simulink library "hapsrav_library"  (R2017a)
settings: Solver=VariableStepAuto  StartTime=0.0  StopTime=10.0  RelTol=1e-3
values from neighbouring files (symbols this model uses):
  absorb_h = 0:100:40000    [EnergySim.m]
  Adisk = pi * v.R_prop^2    [EnergySim.m]
  alpha_h = absorb_h    [EnergySim.m]
  aoa_data = zeros(n_cl, n)    [EnergySim.m]
  cl_bp = linspace(min_cl, max_cl,n_cl)    [EnergySim.m]
  D = [1       -.0065      288.15          0                   101325 ... (first row only)    [EnergySim.m]    (also in msn_params.m = sqrt((from_x - to_x)^2 + (from_y - to_y)^2); solar_vector.m = time.day + ut_time)
  d2r = pi / 180    (= 0.0174532925199)    [EnergySim.m]    (also in example1.m; example2.m; example3.m; example4.m)
  d_init = sqrt(dx*dx + dy*dy)    [EnergySim.m]    (also in msn_init.m)
  dchi0 = atan2(sin(dchi0), cos(dchi0))    [EnergySim.m]    (also in msn_init.m)
  dT = 0.5    [EnergySim.m]
  dT_fixed = 0.5    [EnergySim.m]
  dT_trig = 30    [EnergySim.m]
  earth_rho = 6378137.0    (= 6378137)    [EnergySim.m]
  fp = solarFP(p.orbit_rho, p.min_axis, p.orbit_dir, ic.x_ctr, ic.y_ctr, sun_az_0)    [EnergySim.m]    (also in load_fp.m = gid_tc(msn_idx).fp; solarFP.m = [1	6	2	nul eul 0	0	0	0	1	0)
  fp_coords = [x_entry y_entry]    [msn_params.m]
  fp_courses = [chi_adj nxt_chi dchi]    [msn_params.m]
  g = 9.80665    [EnergySim.m]
  Gsolar = 1367    [EnergySim.m]
  k = k+1    (= 5)    [EnergySim.m]
  K = D(:,2)    [EnergySim.m]
  lat_init = ic.lat_init_deg * obj.d2r    [EnergySim.m]
  M = time.month    [solar_vector.m]
  max_cl = max(cl_data(:))    [EnergySim.m]
  min_cl = min(cl_data(:))    [EnergySim.m]
  ND2 = load(fullfile(pwd,'nd2_data.mat'))    [EnergySim.m]    (also in nd2_data.mat = [0.0999999999999 0.200000000001 0.3 0.4 0.499999999998 0.700)
  next_init = fp(init_wp, 3)    [EnergySim.m]    (also in msn_init.m)
  pE_init = ic.pE_init    [EnergySim.m]
  pN_init = ic.pN_init    [EnergySim.m]
  r2d = 180 / pi    (= 57.2957795131)    [EnergySim.m]    (also in example1.m; example2.m; example3.m; example4.m)
  rho_SL = 1.225    [EnergySim.m]
  S = 110.4    [EnergySim.m]
  thr_lo_lim = 0.0    (= 0)    [EnergySim.m]
  time_init = struct('year', time.year, 'month', time.month,                  'day', time.day, 'hour', time.hour, 'min', time.min,                  'UTC', time.UTC)    [EnergySim.m]
  to_init = fp(init_wp, 1)    [EnergySim.m]    (also in msn_init.m)
  vgnd_init = sqrt(Vg)    [EnergySim.m]
  vtas_init = veas_init * sqrt(rho_sl/rho_alt)    [EnergySim.m]
  w_alt = 2.0 * w_alt    [EnergySim.m]
  w_xtrack = 2.0 * w_xtrack    [EnergySim.m]
undefined symbols (not defined in the file or in its folder): alpha, alpha_bp, alpha_circ, alt0_rate_init, alt_bp, alt_cmd_mode, alt_init, alt_lim_h, alt_lim_l, alt_rt_lim_periodic, cd_data, charge_eff, chi0_rate_init, chi_cmd_mode, chi_inf, chi_init, cl_data, discharge_eff, DiscIntNeverNeededParam, E_batt_max, E_init, Earth, enableFuzzyLogic, entry_init, epsln, epsln_circ, exit_init, f8_azimuth_offset, fig_eight_time, fp0, fp_coords0, fp_courses0, gamma_lim, hold_time, k_c, K_circ, lat_init_deg, lon_init_deg, max_alpha_bp, max_alt_bp, min_alpha_bp, min_alt_bp, min_axis, motor_eff, mppt_eff, num_motors, orb_dir_init, orb_len_init, orbit_dir, orbit_rho, P_acc, panel_eff, panel_vecs, phi_0, phi_lim, phi_lim_alt, phi_lim_alt_max, phi_lim_alt_min, phi_rt_lim, prop_eff_scale ... (+39)
libraries: simulink x59, hapsrav_library x9, fuzblock x3, atmospheric_library x1, aerolibtransform2 x1
(part 3 of 6)

== system hapsrav_library/hapsrav_main/Kinematic 6DOF/Aero/Thrust ==
  d1Vtas : Inport
  gamma : Inport  Port=2
  qS : Inport  Port=3
  CL : Inport  Port=4
  CD : Inport  Port=5
  Display1 : Display
  Display2 : Display
  Display3 : Display
  Divide : Product  Inputs=**
  Divide1 : Product  Inputs=**
  Gain1 : Gain  Gain=M*g
  Gain2 : Gain  Gain=M
  Saturation : Saturate  UpperLimit=9999  LowerLimit=thr_lo_lim
  Sum1 : Sum  Inputs=|++
  Sum5 : Sum  Inputs=|++
  Terminator : Terminator
  Terminator1 : Terminator
  Trigonometric Function : Trigonometry
  thrust : Outport
  wires:
  Saturation/1 -> [thrust]
  Gain1/1 -> Sum1/2
  d1Vtas/1 -> Gain2/1
  Gain2/1 -> Sum1/1
  CL/1 -> Divide/1
  qS/1 -> [qS]
  [qS] -> Divide/2
  Divide/1 -> Display3/1, [lift]
  gamma/1 -> [gamma]
  [gamma] -> Trigonometric Function/1
  Trigonometric Function/1 -> [sin_gamma]
  [sin_gamma] -> Gain1/1
  Sum1/1 -> Sum5/1
  [drag] -> Sum5/2, Display2/1
  [qS] -> Divide1/2
  Divide1/1 -> [drag]
  Sum5/1 -> Display1/1, thrust/1, Saturation/1
  CD/1 -> Divide1/1
  [lift] -> Terminator/1
  [thrust] -> Terminator1/1

== system hapsrav_library/hapsrav_main/Kinematic 6DOF/Airspeed/Std Atmos ==
  alt : Inport
  Constant : Constant  Value=rho_SL
  Divide : Product  Inputs=*/
  NASA-TM-X-74335 Std Atmos 1976 -5 < Alt < 47 km : atmospheric_library/NASA-TM-X-74335 Std Atmos 1976 -5 < Alt < 47 km
  Sqrt : Sqrt  SaturateOnIntegerOverflow=on
  Terminator : Terminator
  rho_ratio : Outport
  OAT : Outport  Port=2
  wires:
  [stat_press] -> Terminator/1
  alt/1 -> NASA-TM-X-74335 Std Atmos 1976 -5 < Alt < 47 km/1
  NASA-TM-X-74335 Std Atmos 1976 -5 < Alt < 47 km/3 -> [rho]
  NASA-TM-X-74335 Std Atmos 1976 -5 < Alt < 47 km/1 -> [OAT]
  NASA-TM-X-74335 Std Atmos 1976 -5 < Alt < 47 km/2 -> [stat_press]
  [OAT] -> OAT/1
  Sqrt/1 -> rho_ratio/1
  Divide/1 -> Sqrt/1
  [rho] -> Divide/2
  Constant/1 -> Divide/1

== system hapsrav_library/hapsrav_main/Kinematic 6DOF/Inertial/East Wind Error ==
  In1 : Inport
  In2 : Inport  Port=2
  In3 : Inport  Port=3
  In4 : Inport  Port=4
  In5 : Inport  Port=5
  In6 : Inport  Port=6
  In7 : Inport  Port=7
  Divide12 : Product  Inputs=***
  Divide13 : Product  Inputs=***
  Sum8 : Sum  Inputs=|+-
  Sum9 : Sum  Inputs=+-|
  We Error : Outport
  wires:
  In4/1 -> Divide12/3
  In2/1 -> Divide12/1
  Divide12/1 -> Sum8/1
  Divide13/1 -> Sum8/2
  In5/1 -> Divide13/1
  In6/1 -> Divide13/2
  In3/1 -> Divide12/2
  In1/1 -> Sum9/1
  Sum9/1 -> We Error/1
  In7/1 -> Divide13/3
  Sum8/1 -> Sum9/2

== system hapsrav_library/hapsrav_main/Kinematic 6DOF/Inertial/Gnd Speed ==
  note: Equation (2.12) of small unmanned aircraft, R. Beard, T. McLain
  Vw2 : Inport
  Vtas : Inport  Port=2
  cos_psi : Inport  Port=3
  cos_ga : Inport  Port=4
  wn : Inport  Port=5
  sin_psi : Inport  Port=6
  we : Inport  Port=7
  sin_ga : Inport  Port=8
  wd : Inport  Port=9
  vgnd0 : Inport  Port=10
  Constant : Constant  Value=0
  Delay2 : Delay  DelayLength=1  InitialConditionSource=Input port
      settings: InputPortMap=u0,p4
  Discrete Differentiator1 : hapsrav_library/Discrete Differentiator
  Divide5 : Product  Inputs=***
  Divide7 : Product  Inputs=***
  Divide8 : Product  Inputs=**
  Divide9 : Product  Inputs=**
  Gain : Gain  Gain=2
  Math Function3 : Math  Operator=square  SaturateOnIntegerOverflow=on
  Sqrt : Sqrt  SaturateOnIntegerOverflow=on
  Sum1 : Sum  Inputs=|++
  Sum4 : Sum  Inputs=+++
  Sum5 : Sum  Inputs=|+-
  Vg : Outport
  d1Vg : Outport  Port=2
  wires:
  Constant/1 -> Discrete Differentiator1/3
  Math Function3/1 -> Sum4/2
  wn/1 -> Divide5/3
  sin_psi/1 -> Divide7/1
  sin_ga/1 -> Divide8/1
  wd/1 -> Divide8/2
  we/1 -> Divide7/3
  cos_psi/1 -> Divide5/1
  Vw2/1 -> Sum4/1
  Gain/1 -> Divide9/1
  Sum4/1 -> Sqrt/1
  Divide9/1 -> Sum4/3
  cos_ga/1 -> [cos_ga]
  [cos_ga] -> Divide5/2
  [cos_ga] -> Divide7/2
  Vtas/1 -> [Vtas]
  [Vtas] -> Gain/1
  [Vtas] -> Math Function3/1
  Divide5/1 -> Sum1/1
  Divide7/1 -> Sum1/2
  Sum1/1 -> Sum5/1
  Divide8/1 -> Sum5/2
  Sum5/1 -> Divide9/2
  Discrete Differentiator1/1 -> d1Vg/1
  Delay2/1 -> Discrete Differentiator1/1, Vg/1
  vgnd0/1 -> Discrete Differentiator1/2, Delay2/2
  Sqrt/1 -> Delay2/1

== system hapsrav_library/hapsrav_main/Kinematic 6DOF/Inertial/Heading ==
  note: Equation (2.11) of small unmanned aircraft, R. Beard, T. McLain
  wn : Inport
  sin_chi : Inport  Port=2
  cos_chi : Inport  Port=3
  we : Inport  Port=4
  Vtas : Inport  Port=5
  cos_ga : Inport  Port=6
  chi : Inport  Port=7
  Divide2 : Product  Inputs=**
  Divide3 : Product  Inputs=**
  Divide4 : Product  Inputs=*/
  Divide6 : Product  Inputs=**
  Sum1 : Sum  Inputs=|-+
  Sum2 : Sum  Inputs=|-+
  Trigonometric Function5 : Trigonometry  Operator=asin
  psi : Outport
  wires:
  we/1 -> Divide3/2
  Divide2/1 -> Sum1/1
  wn/1 -> Divide2/1
  cos_ga/1 -> Divide6/2
  Divide6/1 -> Divide4/2
  Divide4/1 -> Trigonometric Function5/1
  Trigonometric Function5/1 -> Sum2/1
  Divide3/1 -> Sum1/2
  Sum1/1 -> Divide4/1
  Vtas/1 -> Divide6/1
  Sum2/1 -> psi/1
  chi/1 -> Sum2/2
  cos_chi/1 -> Divide3/1
  sin_chi/1 -> Divide2/2

== system hapsrav_library/hapsrav_main/Kinematic 6DOF/Inertial/North Wind Error ==
  In1 : Inport
  In2 : Inport  Port=2
  In3 : Inport  Port=3
  In4 : Inport  Port=4
  In5 : Inport  Port=5
  In6 : Inport  Port=6
  In7 : Inport  Port=7
  Divide10 : Product  Inputs=***
  Divide11 : Product  Inputs=***
  Sum6 : Sum  Inputs=|+-
  Sum7 : Sum  Inputs=+-|
  Wn Error : Outport
  wires:
  In7/1 -> Divide11/3
  In1/1 -> Sum7/1
  Divide10/1 -> Sum6/1
  Divide11/1 -> Sum6/2
  In4/1 -> Divide10/3
  In3/1 -> Divide10/2
  In6/1 -> Divide11/2
  Sum6/1 -> Sum7/2
  In5/1 -> Divide11/1
  In2/1 -> Divide10/1
  Sum7/1 -> Wn Error/1

== system hapsrav_library/hapsrav_main/Kinematic 6DOF/Navigation/Flat Earth to LLA ==
  lat0 : Inport
  lon0 : Inport  Port=2
  pos_N_dot : Inport  Port=3
  pos_E_dot : Inport  Port=4
  alt : Inport  Port=5
  Discrete-Time Integrator : DiscreteIntegrator  IntegratorMethod=Integration: Trapezoidal  InitialConditionSource=external  InitialConditionSetting=State (most efficient)  SampleTime=dT  ICPrevOutput=DiscIntNeverNeededParam  ICPrevScaledInput=DiscIntNeverNeededParam
  Discrete-Time Integrator1 : DiscreteIntegrator  IntegratorMethod=Integration: Trapezoidal  InitialConditionSource=external  InitialConditionSetting=State (most efficient)  SampleTime=dT  ICPrevOutput=DiscIntNeverNeededParam  ICPrevScaledInput=DiscIntNeverNeededParam
  Divide : Product  Inputs=*/
  Divide1 : Product  Inputs=**
  Divide2 : Product  Inputs=*/
  Memory : Memory  X0=lat_init
  Radii of Curvature : Subsystem
  Trigonometric Function1 : Trigonometry  Operator=cos
  wn^1 : Gain  Gain=r2d
  wn^2 : Gain  Gain=r2d
  lat_est : Outport
  lon_est : Outport  Port=2
  wires:
  Radii of Curvature/2(R_M) -> [R_M]
  Radii of Curvature/1(R_N) -> [R_N]
  [lat_est] -> Trigonometric Function1/1
  wn^2/1 -> lat_est/1
  wn^1/1 -> lon_est/1
  [lat_est] -> Memory/1
  Divide/1 -> Discrete-Time Integrator/1
  [R_M] -> Divide/2
  Discrete-Time Integrator/1 -> [lat_est], wn^2/1
  pos_N_dot/1 -> Divide/1
  Discrete-Time Integrator1/1 -> wn^1/1
  pos_E_dot/1 -> Divide2/1
  lat0/1 -> Discrete-Time Integrator/2
  lon0/1 -> Discrete-Time Integrator1/2
  Memory/1 -> Radii of Curvature/1(lat_rad)
  [R_N] -> Divide1/2
  Trigonometric Function1/1 -> Divide1/1
  Divide2/1 -> Discrete-Time Integrator1/1
  Divide1/1 -> Divide2/2
  alt/1 -> [alt]
  [alt] -> Radii of Curvature/2(h)

== system hapsrav_library/hapsrav_main/Kinematic 6DOF/Navigation/Flat Earth to LLA Aero BLockset ==
  alt : Inport
  pN : Inport  Port=2
  pE : Inport  Port=3
  Demux : Demux  Outputs=2
  Flat Earth to LLA : aerolibtransform2/Flat Earth to LLA  units=Metric (MKS)  ptype=Earth (WGS84)  F=1/298.257223563  R=6378137  LL0=[lat_init_deg lon_init_deg]  psi=0
  Mux : Mux  Inputs=3
  Ref Alt : Constant  Value=0
  Terminator : Terminator
  wn^3 : Gain  Gain=-1
  lat_deg : Outport
  lon_deg : Outport  Port=2
  wires:
  wn^3/1 -> Mux/3
  Ref Alt/1 -> Flat Earth to LLA/2
  Mux/1 -> Flat Earth to LLA/1
  alt/1 -> wn^3/1
  pE/1 -> Mux/2
  pN/1 -> Mux/1
  Demux/1 -> lat_deg/1
  Demux/2 -> lon_deg/1
  Flat Earth to LLA/2 -> Terminator/1
  Flat Earth to LLA/1 -> Demux/1

== system hapsrav_library/hapsrav_main/Kinematic 6DOF/Navigation/NED Posn ==
  note: Equation (9.8) of small unmanned aircraft, R. Beard, T. McLain
  Va : Inport
  psi : Inport  Port=2
  we : Inport  Port=3
  wn : Inport  Port=4
  pE0 : Inport  Port=5
  pN0 : Inport  Port=6
  Discrete-Time Integrator : DiscreteIntegrator  IntegratorMethod=Integration: Trapezoidal  InitialConditionSource=external  InitialConditionSetting=State (most efficient)  SampleTime=-1  ICPrevOutput=DiscIntNeverNeededParam  ICPrevScaledInput=DiscIntNeverNeededParam
  Discrete-Time Integrator1 : DiscreteIntegrator  IntegratorMethod=Integration: Trapezoidal  InitialConditionSource=external  InitialConditionSetting=State (most efficient)  SampleTime=-1  ICPrevOutput=DiscIntNeverNeededParam  ICPrevScaledInput=DiscIntNeverNeededParam
  Divide : Product
  Divide1 : Product
  Sum1 : Sum  Inputs=|++
  Sum2 : Sum  Inputs=|++
  Trigonometric Function : Trigonometry
  Trigonometric Function1 : Trigonometry  Operator=cos
  pE : Outport
  pE_dot : Outport  Port=2
  pN : Outport  Port=3
  pN_dot : Outport  Port=4
  wires:
  Divide1/1 -> Sum1/1
  Sum1/1 -> Discrete-Time Integrator1/1, pN_dot/1
  Divide/1 -> Sum2/1
  wn/1 -> Sum1/2
  Sum2/1 -> Discrete-Time Integrator/1, pE_dot/1
  Discrete-Time Integrator1/1 -> pN/1
  psi/1 -> Trigonometric Function/1, Trigonometric Function1/1
  Trigonometric Function/1 -> Divide/1
  Trigonometric Function1/1 -> Divide1/2
  Va/1 -> Divide1/1, Divide/2
  we/1 -> Sum2/2
  Discrete-Time Integrator/1 -> pE/1
  pE0/1 -> Discrete-Time Integrator/2
  pN0/1 -> Discrete-Time Integrator1/2

== system hapsrav_library/hapsrav_main/Kinematic 6DOF/Power Model/Battery and Potential Management ==
  note: P (kW)
  P_el_in : Inport
  P_el_out : Inport  Port=2
  alt : Inport  Port=3
  hdot : Inport  Port=4
  1/discharge_eff : Gain  Gain=1/discharge_eff
  Climb Rate : Subsystem
  Constant : Constant  Value=E_init
  Constant1 : Constant  Value=alt_lim_l
  Constant3 : Constant  Value=0
  Delay1 : Delay  DelayLength=1  InitialConditionSource=Input port  InitialCondition=E_init
      settings: InputPortMap=u0,p4
  Discrete-Time Integrator1 : DiscreteIntegrator  IntegratorMethod=Integration: Trapezoidal  InitialCondition=E_init  InitialConditionSetting=State (most efficient)  SampleTime=-1  ICPrevOutput=DiscIntNeverNeededParam  ICPrevScaledInput=DiscIntNeverNeededParam
  Gain2 : Gain  Gain=M*g
  Gain4 : Gain  Gain=M*g
  Multiport Switch : MultiPortSwitch  DataPortOrder=Specify indices  DataPortIndices={-1, 0, 1}
  Stateflow Battery Management : Stateflow chart  TreatAsAtomicUnit=on
  Stateflow Potential Management : Stateflow chart  TreatAsAtomicUnit=on
  Sum{,1..3} (4 alike) : Sum  Inputs=|+-
  W to kW1 : Gain  Gain=0.001
  W to kW2 : Gain  Gain=0.001
  charge_eff : Gain  Gain=charge_eff
  to kWh1 : Gain  Gain=1/(60*60)
  to kWh2 : Gain  Gain=1/(60*60)
  powered_climb_rt : Outport
  E_batt : Outport  Port=2
  P_batt : Outport  Port=3
  E_gravit : Outport  Port=4
  charge_mode : Outport  Port=5
  climb_mode : Outport  Port=6
  wires:
  Sum/1 -> [P_el_net]
  to kWh1/1 -> E_gravit/1
  [P_el_net] -> Stateflow Battery Management/1(P_el_net)
  Stateflow Battery Management/1(ChargeMode) -> charge_mode/1, Multiport Switch/1
  to kWh2/1 -> Discrete-Time Integrator1/1
  Multiport Switch/1 -> P_batt/1, to kWh2/1  "P_batt"
  Discrete-Time Integrator1/1 -> Delay1/1, E_batt/1
  charge_eff/1 -> Multiport Switch/4
  Constant3/1 -> Multiport Switch/3
  1/discharge_eff/1 -> Multiport Switch/2
  [P_el_net] -> charge_eff/1, 1/discharge_eff/1
  [P_el_in] -> Stateflow Potential Management/4(P_el_in)
  [P_el_out] -> Sum1/1
  Gain2/1 -> W to kW2/1
  W to kW2/1 -> Sum1/2
  Sum1/1 -> [P_cruise]
  [P_cruise] -> Stateflow Potential Management/1(P_cruise)
  [P_el_in] -> Sum2/1
  [P_cruise] -> Sum2/2
  Sum2/1 -> [P_el_net_cruise]
  Stateflow Potential Management/1(ClimbMode) -> climb_mode/1, Climb Rate/1(ClimbMode)
  hdot/1 -> [hdot]
  P_el_in/1 -> [P_el_in]
  P_el_out/1 -> [P_el_out]
  alt/1 -> [alt]
  [P_el_out] -> Sum/2
  [P_el_in] -> Sum/1
  [hdot] -> Gain2/1
  [alt] -> Stateflow Potential Management/2(alt)
  Climb Rate/1(powered_climb_rt) -> powered_climb_rt/1
  [P_el_net] -> Climb Rate/4(P_el_net)
  [P_el_net_cruise] -> Climb Rate/3(P_el_net_cruise)
  [P_el_out] -> Climb Rate/2(P_el_out)
  Delay1/1 -> Stateflow Potential Management/3(E_batt), Stateflow Battery Management/2(E_batt)
  Constant/1 -> Delay1/2
  W to kW1/1 -> to kWh1/1
  Gain4/1 -> W to kW1/1
  [alt] -> Sum3/1
  Sum3/1 -> Gain4/1
  Constant1/1 -> Sum3/2

== system hapsrav_library/hapsrav_main/Kinematic 6DOF/Power Model/Electric Power In ==
  sun_az : Inport
  sun_zth : Inport  Port=2
  julian_day : Inport  Port=3
  vehicle_yaw : Inport  Port=4
  vehicle_pitch : Inport  Port=5
  vehicle_roll : Inport  Port=6
  alt : Inport  Port=7
  trigger : Inport  Port=8
  Delay : Delay  DelayLength=1  InitialCondition=0
  Demux : Demux  Outputs=[1 1 1]
  Discrete-Time Integrator : DiscreteIntegrator  IntegratorMethod=Integration: Trapezoidal  InitialConditionSetting=State (most efficient)  SampleTime=-1  ICPrevOutput=DiscIntNeverNeededParam  ICPrevScaledInput=DiscIntNeverNeededParam
  Discrete-Time Integrator1 : DiscreteIntegrator  IntegratorMethod=Integration: Trapezoidal  InitialConditionSetting=State (most efficient)  SampleTime=-1  ICPrevOutput=DiscIntNeverNeededParam  ICPrevScaledInput=DiscIntNeverNeededParam
  MPPT efficiency : Gain  Gain=mppt_eff
  Terminator1 : Terminator
  Terminator2 : Terminator
  W to KW : Gain  Gain=0.001
  atmos_absorb_adj : Subsystem  TreatAsAtomicUnit=on
  non negative1 : Saturate  UpperLimit=9e99  LowerLimit=0
  panel efficiency : Gain  Gain=panel_eff
  pow_calc : Product
  pow_calc1 : Product  Inputs=3
  pow_calc2 : Product
  projected area : Subsystem
  solar constant : Constant  Value=Gsolar
  solar_dist_adj : Subsystem  TreatAsAtomicUnit=on
  solar_vec_ned : Subsystem  TreatAsAtomicUnit=on
  to kWh : Gain  Gain=1/(60*60)
  to kWh1 : Gain  Gain=1/(60*60)
  P_el_in : Outport
  E_el_in : Outport  Port=2
  projected_area : Outport  Port=3
  G_adjusted : Outport  Port=4
  E_solar_flat : Outport  Port=5
  wires:
  pow_calc/1 -> W to KW/1
  W to KW/1 -> panel efficiency/1
  sun_az/1 -> solar_vec_ned/1(az)  "deg"
  sun_zth/1 -> solar_vec_ned/2(zth), atmos_absorb_adj/1(sun_zth)  "deg"
  panel efficiency/1 -> MPPT efficiency/1
  Discrete-Time Integrator/1 -> E_el_in/1
  to kWh/1 -> Discrete-Time Integrator/1
  julian_day/1 -> solar_dist_adj/1(jd)
  vehicle_yaw/1 -> projected area/1(yaw)  "deg"
  vehicle_pitch/1 -> projected area/2(pitch)  "deg"
  vehicle_roll/1 -> projected area/3(roll)  "deg"
  solar_vec_ned/1(sun_ned) -> projected area/4(sun), Demux/1
  projected area/1(projected_area) -> projected_area/1, pow_calc/1  "projected area (m2)"
  atmos_absorb_adj/1(atmos_adj) -> pow_calc1/2
  pow_calc1/1 -> G_adjusted/1, pow_calc2/2, pow_calc/2
  alt/1 -> atmos_absorb_adj/2(altitude)
  trigger/1 -> Delay/1
  Delay/1 -> [trigger]
  [trigger] -> solar_vec_ned/Trigger
  [trigger] -> solar_dist_adj/Trigger
  [trigger] -> atmos_absorb_adj/Trigger
  solar_dist_adj/1(dist_adj) -> pow_calc1/3
  solar constant/1 -> pow_calc1/1
  MPPT efficiency/1 -> to kWh/1, P_el_in/1
  Demux/3 -> non negative1/1
  pow_calc2/1 -> to kWh1/1
  to kWh1/1 -> Discrete-Time Integrator1/1
  non negative1/1 -> pow_calc2/1
  Discrete-Time Integrator1/1 -> E_solar_flat/1
  Demux/2 -> Terminator2/1
  Demux/1 -> Terminator1/1

== system hapsrav_library/hapsrav_main/Kinematic 6DOF/Power Model/Electric Power Out ==
  P_acc : Inport
  vtas : Inport  Port=2
  thrust : Inport  Port=3
  qbar : Inport  Port=4
  Discrete-Time Integrator1 : DiscreteIntegrator  IntegratorMethod=Integration: Trapezoidal  InitialConditionSetting=State (most efficient)  SampleTime=-1  ICPrevOutput=DiscIntNeverNeededParam  ICPrevScaledInput=DiscIntNeverNeededParam
  Divide : Product  Inputs=*/
  Product : Product
  Sum : Sum  Inputs=|++
  W to KW : Gain  Gain=0.001
  motor eff : Gain  Gain=motor_eff
  non negative : Saturate  UpperLimit=9e99  LowerLimit=0
  "prop_eff (theoretical max from actuator disk theory, scaled by coeff < 1) (http://web.mit.edu/16.unified/www/FALL/thermodynamics/notes/node86.html)" : Subsystem
  to kWh : Gain  Gain=1/3600
  P_el_out : Outport
  E_el_out : Outport  Port=2
  prop_eff : Outport  Port=3
  wires:
  P_acc/1 -> Sum/1
  vtas/1 -> Product/1
  Divide/1 -> non negative/1
  Sum/1 -> W to KW/1
  qbar/1 -> "prop_eff (theoretical max from actuator disk theory, scaled by coeff < 1) (http://web.mit.edu/16.unified/www/FALL/thermodynamics/notes/node86.html)"/2(qbar)
  "prop_eff (theoretical max from actuator disk theory, scaled by coeff < 1) (http://web.mit.edu/16.unified/www/FALL/thermodynamics/notes/node86.html)"/1(prop_eff) -> motor eff/1, prop_eff/1
  non negative/1 -> Sum/2
  to kWh/1 -> Discrete-Time Integrator1/1
  W to KW/1 -> to kWh/1, P_el_out/1
  thrust/1 -> Product/2, "prop_eff (theoretical max from actuator disk theory, scaled by coeff < 1) (http://web.mit.edu/16.unified/www/FALL/thermodynamics/notes/node86.html)"/1(thrust)
  Discrete-Time Integrator1/1 -> E_el_out/1
  motor eff/1 -> Divide/2
  Product/1 -> Divide/1

== system hapsrav_library/hapsrav_main/Kinematic 6DOF/Power Model/sun_position ==
  lon : Inport
  lat : Inport  Port=2
  alt : Inport  Port=3
  clock : Inport  Port=4
  Trigger : TriggerPort  TriggerType=either  VariantControl=Variant  InitialTriggerSignalState=positive
  Constant : Constant  Value=time_init
  Constant1 : Constant  Value=90
  Demux : Demux  Outputs=6
  Floor1 : Rounding
  Sum : Sum  Inputs=|+-
  UTC : Constant  Value=UTC
  sun_pos : MATLAB Function  TreatAsAtomicUnit=on
  time_update : MATLAB Function  TreatAsAtomicUnit=on
  sun_az : Outport
  sun_zth : Outport  Port=2
  jd : Outport  Port=3
  sun_el : Outport  Port=4
  wires:
  sun_pos/1(sun_az) -> sun_az/1
  sun_pos/2(sun_zth) -> sun_zth/1, Sum/2
  Floor1/1 -> time_update/2(sim_secs)
  sun_pos/3(jd) -> jd/1
  Demux/3 -> sun_pos/3(t3)
  lon/1 -> sun_pos/8(l1)
  Demux/1 -> sun_pos/1(t1)
  Demux/4 -> sun_pos/4(t4)
  lat/1 -> sun_pos/9(l2)
  Constant/1 -> time_update/1(time_init)
  alt/1 -> sun_pos/10(l3)
  clock/1 -> Floor1/1  "since_init"
  Demux/5 -> sun_pos/5(t5)
  Demux/2 -> sun_pos/2(t2)
  Demux/6 -> sun_pos/6(t6)
  UTC/1 -> sun_pos/7(t7)
  time_update/1(t_new) -> Demux/1
  Constant1/1 -> Sum/1
  Sum/1 -> sun_el/1

== system hapsrav_library/hapsrav_main/Kinematic 6DOF/Selectable Modes/Trajectory_Optimization ==
  vert_lat_cmds : Inport
  Vg : Inport  Port=2
  s6dof0 : Inport  Port=3
  max_clmb_rt : Inport  Port=4
  max_desc_rt : Inport  Port=5
  idleDesc : Inport  Port=6
  Enable : EnablePort
  Altitude : Subsystem
  Bus Selector : BusSelector  OutputSignals=alt0,chi0,altRt0,phi0
  Demux : Demux  Outputs=2
  Lat Cmd Filter : Subsystem
  Roll : Subsystem
  Vert Cmd Filter : Subsystem
  alt : Outport
  d1alt : Outport  Port=2
  phi : Outport  Port=3
  chi : Outport  Port=4
  wires:
  [neg_vv_lim] -> Vert Cmd Filter/4(lolim)
  [pos_vv_lim] -> Vert Cmd Filter/3(uplim)
  [neg_vv_lim] -> Altitude/3(max_desc_rt)
  [pos_vv_lim] -> Altitude/2(max_clmb_rt)
  max_desc_rt/1 -> [neg_vv_lim]
  max_clmb_rt/1 -> [pos_vv_lim]
  Roll/2(chi) -> [chi]
  idleDesc/1 -> Altitude/6(idleDesc)
  [chi] -> chi/1
  [phi] -> phi/1
  [d1alt] -> d1alt/1
  [alt] -> alt/1
  Roll/1(roll) -> [phi]
  [roll_cmd] -> Lat Cmd Filter/1(roll cmd)
  Lat Cmd Filter/1(filt roll cmd) -> [filtRollCmd]
  [roll0] -> Lat Cmd Filter/2(roll0)
  Vg/1 -> [Vg]
  Altitude/1(alt) -> [alt]
  Altitude/2(d1alt) -> [d1alt]
  [filtAltRtCmd] -> Altitude/1(altRt_cmd)
  Demux/2 -> [roll_cmd]
  [hdot_cmd] -> Vert Cmd Filter/1(hdot_cmd)
  Demux/1 -> [hdot_cmd]
  [alt_rt_0] -> Vert Cmd Filter/2(altRt0)
  Vert Cmd Filter/1(filt hdot cmd) -> [filtAltRtCmd]
  vert_lat_cmds/1 -> Demux/1
  [alt_rt_0] -> Altitude/5(altRt0)
  [Vg] -> Roll/4(Vg)
  [alt] -> Roll/3(alt)
  [roll0] -> Roll/2(roll0)
  [filtRollCmd] -> Roll/1(filtRollcmd)
  s6dof0/1 -> Bus Selector/1
  Bus Selector/1 -> [alt0]  "<alt0>"
  [alt0] -> Altitude/4(alt0)
  Bus Selector/2 -> [chi0]  "<chi0>"
  [chi0] -> Roll/5(chi0)
  Bus Selector/4 -> [roll0]  "<phi0>"
  Bus Selector/3 -> [alt_rt_0]  "<altRt0>"

== system hapsrav_library/hapsrav_main/Kinematic 6DOF/Selectable Modes/Waypoint_Navigation ==
  vert_lat_cmds : Inport
  Vg : Inport  Port=2
  d1Vg : Inport  Port=3
  s6dof0 : Inport  Port=4
  max_clmb_rt : Inport  Port=5
  max_desc_rt : Inport  Port=6
  idleDesc : Inport  Port=7
  Enable : EnablePort
  Altitude : Subsystem
  Bus Selector : BusSelector  OutputSignals=alt0,chi0,altRt0
  Course : Subsystem
  Demux : Demux  Outputs=2
  Lat Cmd Filter : Subsystem
  Vert Cmd Filter : Subsystem
  alt : Outport
  d1alt : Outport  Port=2
  phi : Outport  Port=3
  chi : Outport  Port=4
  wires:
  Lat Cmd Filter/1(filt chi cmd) -> [filtChiCmd]
  [chi_cmd] -> Lat Cmd Filter/1(chi cmd)
  [max_desc_rt] -> Altitude/4(max_desc_rt)
  [max_clmb_rt] -> Altitude/3(max_clmb_rt)
  [max_desc_rt] -> Vert Cmd Filter/4(max_desc_rt)
  [max_clmb_rt] -> Vert Cmd Filter/3(max_clmb_rt)
  max_desc_rt/1 -> [max_desc_rt]
  max_clmb_rt/1 -> [max_clmb_rt]
  idleDesc/1 -> Altitude/6(idleDesc)
  [alt_rt_0] -> Altitude/5(alt_rt_init)
  Bus Selector/3 -> [alt_rt_0]  "<altRt0>"
  vert_lat_cmds/1 -> Demux/1
  Vert Cmd Filter/1(filt alt cmd) -> [filtAltCmd]
  [alt0] -> Vert Cmd Filter/2(alt_init)
  Demux/1 -> [alt_cmd]
  [alt_cmd] -> Vert Cmd Filter/1(alt cmd)
  Demux/2 -> [chi_cmd]
  [filtAltCmd] -> Altitude/1(alt_cmd)
  [alt0] -> Altitude/2(alt0)
  Altitude/2(d1alt) -> [d1alt]
  Altitude/1(alt) -> [alt]
  Vg/1 -> [Vg]
  [chi0] -> Lat Cmd Filter/2(chi_init)
  Course/2(chi) -> [chi]
  [Vg] -> Course/1(Vg)
  [chi0] -> Course/4(chi0)
  [filtChiCmd] -> Course/3(chi_cmd)
  Course/1(phi) -> [phi]
  [alt] -> Course/2(alt)
  d1Vg/1 -> [d1Vg]
  [d1Vg] -> Course/5(d1Vg)
  [alt] -> alt/1
  [d1alt] -> d1alt/1
  [phi] -> phi/1
  [chi] -> chi/1
  s6dof0/1 -> Bus Selector/1
  Bus Selector/1 -> [alt0]  "<alt0>"
  Bus Selector/2 -> [chi0]  "<chi0>"

== system hapsrav_library/Cmd - Parametric/Chi Cmd/Flight Plan/D2N/Distance ==
  to_x : Inport
  from_x : Inport  Port=2
  to_y : Inport  Port=3
  from_y : Inport  Port=4
  Product of Elements : Product
  Product of Elements1 : Product
  Sqrt : Sqrt  SaturateOnIntegerOverflow=on
  Sum : Sum  Inputs=|+-
  Sum1 : Sum  Inputs=|+-
  Sum2 : Sum  Inputs=|++
  Dist : Outport
  wires:
  Sum1/1 -> [dy]
  to_x/1 -> Sum/1
  Sum/1 -> [dx]
  from_y/1 -> Sum1/2
  to_y/1 -> Sum1/1
  Sqrt/1 -> Dist/1
  Sum2/1 -> Sqrt/1
  [dx] -> Product of Elements/1, Product of Elements/2
  Product of Elements1/1 -> Sum2/2
  Product of Elements/1 -> Sum2/1
  [dy] -> Product of Elements1/1, Product of Elements1/2
  from_x/1 -> Sum/2

== system hapsrav_library/Cmd - Parametric/Chi Cmd/Flight Plan/Mission Command/Entry Mode ==
  leg_state : Inport
  av_state : Inport  Port=2
  Enable : EnablePort  StatesWhenEnabling=reset
  Bus Selector1 : BusSelector  OutputSignals=av_posn,av_course,av_gndspeed
  Constant1 : Constant  Value=alpha
  Constant2 : Constant  Value=epsln
  Constant3 : Constant  Value=k
  Constant4 : Constant  Value=K
  Constant5 : Constant  Value=chi_inf
  Constant6 : Constant  Value=0
  Desired Course : Subsystem  TreatAsAtomicUnit=on
  Desired Course1 : Subsystem  TreatAsAtomicUnit=on
  Logical Operator : Logic  Operator=NOT  Inputs=1  AllPortsSameDT=off  OutDataTypeStr=boolean
  MATLAB Function : MATLAB Function  TreatAsAtomicUnit=on
  Merge : Merge
  xtrack Error : Subsystem  TreatAsAtomicUnit=on
  chi_cmd : Outport
  chi_d : Outport  Port=2
  xtrack : Outport  Port=3
  sweep : Outport  Port=4
  wires:
  [av_posn] -> Desired Course1/2(av_posn)
  [av_posn] -> xtrack Error/2(av_posn)
  Bus Selector1/1 -> [av_posn]  "<av_posn>"
  [leg_state] -> Desired Course1/1(leg_state)
  [leg_state] -> xtrack Error/1(leg_state)
  leg_state/1 -> [leg_state]
  Merge/1 -> [chi_d]
  [chi_d_1] -> Merge/2
  [chi_d_0] -> Merge/1
  [collocated] -> Desired Course1/Enable
  Desired Course1/1(chi_d) -> [chi_d_1]
  Logical Operator/1 -> Desired Course/Enable
  [collocated] -> Logical Operator/1
  xtrack Error/3(collocated) -> [collocated]
  Constant6/1 -> sweep/1
  Bus Selector1/3 -> [Vg]  "<av_gndspeed>"
  av_state/1 -> Bus Selector1/1
  Bus Selector1/2 -> [chi]  "<av_course>"
  [chi_d] -> chi_d/1
  Desired Course/1(chi_d) -> [chi_d_0]
  [Vg] -> MATLAB Function/4(Vg)
  [chi] -> MATLAB Function/1(chi)
  Constant5/1 -> MATLAB Function/5(chi_inf)
  Constant3/1 -> MATLAB Function/8(k)
  [chi_d] -> MATLAB Function/2(chi_d)
  [xtrack] -> MATLAB Function/3(xtrack)
  Constant2/1 -> MATLAB Function/7(e)
  Constant1/1 -> MATLAB Function/6(alpha)
  Constant4/1 -> MATLAB Function/9(K)
  MATLAB Function/1(chi_cmd) -> chi_cmd/1
  [xtrack] -> Desired Course/2(xtrack)
  [leg_crs] -> Desired Course/1(leg_crs)
  [xtrack] -> xtrack/1
  xtrack Error/2(xtrk) -> [xtrack]
  xtrack Error/1(leg_crs) -> [leg_crs]

== system hapsrav_library/Cmd - Parametric/Chi Cmd/Flight Plan/Mission Command/Not Entry Mode ==
  orbit_state : Inport
  leg_state : Inport  Port=2
  av_state : Inport  Port=3
  nav_mode : Inport  Port=4
  Enable : EnablePort  StatesWhenEnabling=reset
  Circular Pattern Holding : Subsystem
  Compare To Constant : simulink/Logic and Bit Operations/Compare To Constant  relop===  const=3  OutDataTypeStr=boolean
  Compare To Constant3 : simulink/Logic and Bit Operations/Compare To Constant  relop=~=  const=3  OutDataTypeStr=boolean
  Linear Following : Subsystem  TreatAsAtomicUnit=on
  Merge{,1..3} (4 alike) : Merge
  chi_cmd : Outport
  chi_d : Outport  Port=2
  xtrack : Outport  Port=3
  sweep : Outport  Port=4
  wires:
  Merge3/1 -> sweep/1
  [sweep_3] -> Merge3/2
  [sweep_2] -> Merge3/1
  Circular Pattern Holding/4(sweep) -> [sweep_3]
  Linear Following/4(sweep) -> [sweep_2]
  orbit_state/1 -> Circular Pattern Holding/2(orbit_state)
  Linear Following/1(chi_cmd) -> [chi_cmd_2]
  Linear Following/2(chi_d) -> [chi_d_2]
  Linear Following/3(xtrack) -> [xtrack_2]
  Compare To Constant3/1 -> Linear Following/Enable
  [nav_mode] -> Compare To Constant3/1
  [av_state] -> Linear Following/2(av_state)
  [leg_state] -> Linear Following/1(leg_state)
  nav_mode/1 -> [nav_mode]
  Compare To Constant/1 -> Circular Pattern Holding/Enable
  [xtrack_3] -> Merge2/2
  [xtrack_2] -> Merge2/1
  [chi_d_3] -> Merge1/2
  [chi_d_2] -> Merge1/1
  [chi_cmd_3] -> Merge/2
  [chi_cmd_2] -> Merge/1
  Circular Pattern Holding/3(xtrack) -> [xtrack_3]
  Circular Pattern Holding/2(chi_d) -> [chi_d_3]
  Circular Pattern Holding/1(chi_cmd) -> [chi_cmd_3]
  [av_state] -> Circular Pattern Holding/1(av_state)
  [nav_mode] -> Compare To Constant/1
  av_state/1 -> [av_state]
  leg_state/1 -> [leg_state]
  Merge2/1 -> xtrack/1
  Merge1/1 -> chi_d/1
  Merge/1 -> chi_cmd/1

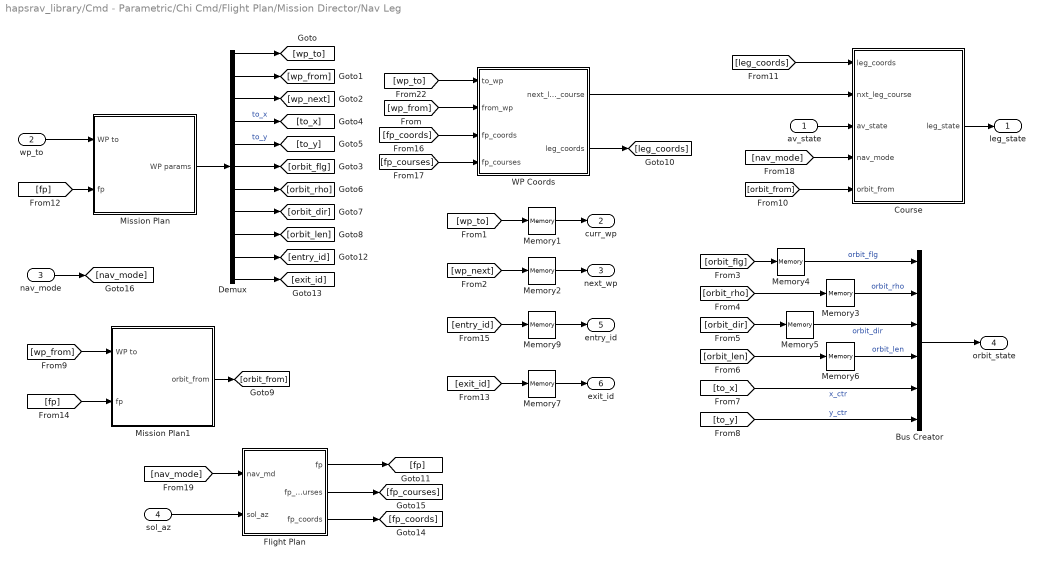
== system hapsrav_library/Cmd - Parametric/Chi Cmd/Flight Plan/Mission Director/Nav Leg ==
  av_state : Inport
  wp_to : Inport  Port=2
  nav_mode : Inport  Port=3
  sol_az : Inport  Port=4
  Bus Creator : BusCreator  Inputs='orbit_flg','orbit_rho','orbit_dir','orbit_len','x_ctr','y_ctr'
  Course : Subsystem
  Demux : Demux  Outputs=11
  Flight Plan : Subsystem
  Memory1 : Memory  X0=to_init
  Memory2 : Memory  X0=next_init
  Memory3 : Memory
  Memory4 : Memory
  Memory5 : Memory  X0=orb_dir_init
  Memory6 : Memory  X0=orb_len_init
  Memory7 : Memory  X0=exit_init
  Memory9 : Memory  X0=entry_init
  Mission Plan : Subsystem
  Mission Plan1 : Subsystem
  WP Coords : Subsystem
  leg_state : Outport
  curr_wp : Outport  Port=2
  next_wp : Outport  Port=3
  orbit_state : Outport  Port=4
  entry_id : Outport  Port=5
  exit_id : Outport  Port=6
  wires:
  sol_az/1 -> Flight Plan/2(sol_az)
  Flight Plan/3(fp_coords) -> [fp_coords]
  Flight Plan/2(fp_courses) -> [fp_courses]
  [nav_mode] -> Flight Plan/1(nav_md)
  [nav_mode] -> Course/4(nav_mode)
  nav_mode/1 -> [nav_mode]
  [fp_courses] -> WP Coords/4(fp_courses)
  [fp_coords] -> WP Coords/3(fp_coords)
  [fp] -> Mission Plan1/2(fp)
  [fp] -> Mission Plan/2(fp)
  Flight Plan/1(fp) -> [fp]
  WP Coords/1(next_leg_course) -> Course/2(nxt_leg_course)
  [exit_id] -> Memory7/1
  Memory7/1 -> exit_id/1
  Demux/11 -> [exit_id]
  Memory9/1 -> entry_id/1
  [entry_id] -> Memory9/1
  Demux/10 -> [entry_id]
  [leg_coords] -> Course/1(leg_coords)
  WP Coords/2(leg_coords) -> [leg_coords]
  [orbit_from] -> Course/5(orbit_from)
  [wp_from] -> Mission Plan1/1(WP to)
  Mission Plan1/1(orbit_from) -> [orbit_from]
  Mission Plan/1(WP params) -> Demux/1
  wp_to/1 -> Mission Plan/1(WP to)
  [to_y] -> Bus Creator/6  "y_ctr"
  [to_x] -> Bus Creator/5  "x_ctr"
  Demux/5 -> [to_y]  "to_y"
  Demux/4 -> [to_x]  "to_x"
  Course/1(leg_state) -> leg_state/1
  [wp_from] -> WP Coords/2(from_wp)
  [wp_to] -> WP Coords/1(to_wp)
  Memory5/1 -> Bus Creator/3  "orbit_dir"
  Memory3/1 -> Bus Creator/2  "orbit_rho"
  Memory4/1 -> Bus Creator/1  "orbit_flg"
  Memory6/1 -> Bus Creator/4  "orbit_len"
  Memory2/1 -> next_wp/1
  Memory1/1 -> curr_wp/1
  av_state/1 -> Course/3(av_state)
  Bus Creator/1 -> orbit_state/1
  [orbit_len] -> Memory6/1
  [orbit_flg] -> Memory4/1
  Demux/6 -> [orbit_flg]
  [orbit_dir] -> Memory5/1
  [orbit_rho] -> Memory3/1
  [wp_next] -> Memory2/1
  [wp_to] -> Memory1/1
  Demux/1 -> [wp_to]
  Demux/7 -> [orbit_rho]
  Demux/3 -> [wp_next]
  Demux/2 -> [wp_from]
  Demux/8 -> [orbit_dir]
  Demux/9 -> [orbit_len]

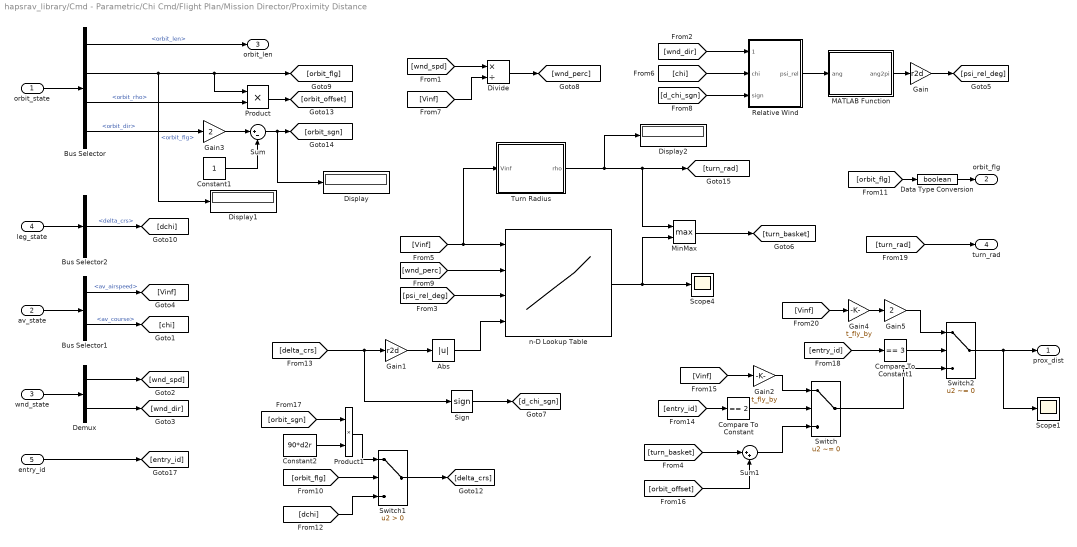
== system hapsrav_library/Cmd - Parametric/Chi Cmd/Flight Plan/Mission Director/Proximity Distance ==
  orbit_state : Inport
  av_state : Inport  Port=2
  wnd_state : Inport  Port=3
  leg_state : Inport  Port=4
  entry_id : Inport  Port=5
  Abs : Abs
  Bus Selector : BusSelector  OutputSignals=orbit_len,orbit_flg,orbit_rho,orbit_dir
  Bus Selector1 : BusSelector  OutputSignals=av_airspeed,av_course
  Bus Selector2 : BusSelector  OutputSignals=crs_state.delta_crs
  Compare To Constant : simulink/Logic and Bit Operations/Compare To Constant  relop===  const=2  OutDataTypeStr=boolean
  Compare To Constant1 : simulink/Logic and Bit Operations/Compare To Constant  relop===  const=3  OutDataTypeStr=boolean
  Constant1 : Constant
  Constant2 : Constant  Value=90*d2r
  Data Type Conversion : DataTypeConversion  OutDataTypeStr=boolean
  Demux : Demux  Outputs=2
  Display : Display
  Display1 : Display
  Display2 : Display
  Divide : Product  Inputs=*/
  Gain : Gain  Gain=r2d
  Gain1 : Gain  Gain=r2d
  Gain2 : Gain  Gain=t_fly_by
  Gain3 : Gain  Gain=2
  Gain4 : Gain  Gain=t_fly_by
  Gain5 : Gain  Gain=2
  MATLAB Function : MATLAB Function  TreatAsAtomicUnit=on
  MinMax : MinMax  Function=max  Inputs=2
  Product : Product
  Product1 : Product
  Relative Wind : Subsystem
  Scope1 : Scope
  Scope4 : Scope
  Sign : Signum
  Sum : Sum  Inputs=|+-
  Sum1 : Sum  Inputs=|++
  Switch : Switch  Criteria=u2 ~= 0
  Switch1 : Switch  Criteria=u2 > Threshold
  Switch2 : Switch  Criteria=u2 ~= 0
  Turn Radius : Subsystem
  n-D Lookup Table : Lookup_n-D  NumberOfTableDimensions=4  BreakpointsForDimension1="[10 20 30  40  50  70  80  90  100 120 140]"  BreakpointsForDimension2=[0 0.1 0.2 0.3 0.4 0.5 0.6 0.7 0.8]  BreakpointsForDimension3=[0:30:360]  BreakpointsForDimension4=[0:5:175]  IndexSearchMethod=Linear search  BeginIndexSearchUsingPreviousIndexResult=on  Table=ND2  ExtrapMethod=Clip  DiagnosticForOutOfRangeInput=Warning  UseLastTableValue=on  InternalRulePriority=Speed  RndMeth=Simplest  InputSameDT=on
  prox_dist : Outport
  orbit_flg : Outport  Port=2
  orbit_len : Outport  Port=3
  turn_rad : Outport  Port=4
  wires:
  Compare To Constant/1 -> Switch/2
  Compare To Constant1/1 -> Switch2/2
  [entry_id] -> Compare To Constant1/1
  [entry_id] -> Compare To Constant/1
  entry_id/1 -> [entry_id]
  Data Type Conversion/1 -> orbit_flg/1
  Gain5/1 -> Switch2/1
  Gain4/1 -> Gain5/1
  [Vinf] -> Gain4/1
  Switch/1 -> Switch2/3
  Switch2/1 -> prox_dist/1, Scope1/1
  [psi_rel_deg] -> n-D Lookup Table/3
  [wnd_perc] -> n-D Lookup Table/2
  [turn_rad] -> turn_rad/1
  Demux/1 -> [wnd_spd]
  Demux/2 -> [wnd_dir]
  Bus Selector/3 -> Product/2  "<orbit_rho>"
  [orbit_sgn] -> Product1/1
  Product1/1 -> Switch1/1
  Constant2/1 -> Product1/2
  Constant1/1 -> Sum/2
  Sum/1 -> [orbit_sgn], Display/1
  Gain3/1 -> Sum/1
  Bus Selector/4 -> Gain3/1  "<orbit_dir>"
  [dchi] -> Switch1/3
  Switch1/1 -> [delta_crs]
  [orbit_flg] -> Switch1/2
  [orbit_flg] -> Data Type Conversion/1
  MinMax/1 -> [turn_basket]
  Sum1/1 -> Switch/3
  [orbit_offset] -> Sum1/2
  [turn_basket] -> Sum1/1
  Gain2/1 -> Switch/1
  [Vinf] -> Gain2/1
  [delta_crs] -> Gain1/1, Sign/1
  Bus Selector2/1 -> [dchi]  "<delta_crs>"
  leg_state/1 -> Bus Selector2/1
  n-D Lookup Table/1 -> MinMax/2, Scope4/1
  Relative Wind/1(psi_rel) -> MATLAB Function/1(ang)
  [d_chi_sgn] -> Relative Wind/3(sign)
  [chi] -> Relative Wind/2(chi)
  [wnd_dir] -> Relative Wind/1(wind_dir)
  Sign/1 -> [d_chi_sgn]
  Divide/1 -> [wnd_perc]
  [Vinf] -> Divide/2
  [wnd_spd] -> Divide/1
  Abs/1 -> n-D Lookup Table/4
  Bus Selector1/2 -> [chi]  "<av_course>"
  Gain1/1 -> Abs/1
  Turn Radius/1(rho) -> MinMax/1, [turn_rad], Display2/1
  Gain/1 -> [psi_rel_deg]
  MATLAB Function/1(ang2pi) -> Gain/1
  wnd_state/1 -> Demux/1
  [Vinf] -> n-D Lookup Table/1, Turn Radius/1(Vinf)
  Bus Selector1/1 -> [Vinf]  "<av_airspeed>"
  av_state/1 -> Bus Selector1/1
  Product/1 -> [orbit_offset]
  Bus Selector/2 -> Product/1, [orbit_flg], Display1/1  "<orbit_flg>"
  Bus Selector/1 -> orbit_len/1  "<orbit_len>"
  orbit_state/1 -> Bus Selector/1

== system hapsrav_library/Cmd - Parametric/Chi Cmd/Flight Plan/Mission Director/Sweep Logic ==
  exit_id : Inport
  sweep : Inport  Port=2
  orbit_len : Inport  Port=3
  Compare To Constant : simulink/Logic and Bit Operations/Compare To Constant  relop===  const=5  OutDataTypeStr=boolean
  Constant : Constant  Value=3*d2r
  Gain : Gain  Gain=d2r
  Logical Operator : Logic  AllPortsSameDT=off  OutDataTypeStr=boolean
  Memory6 : Memory
  Relational Operator : RelationalOperator  Operator=<=  OutDataTypeStr=boolean  RndMeth=Simplest
  Sum : Sum  Inputs=|++
  sweep_flg : Outport
  wires:
  Gain/1 -> Relational Operator/2
  Logical Operator/1 -> sweep_flg/1
  exit_id/1 -> Compare To Constant/1
  orbit_len/1 -> Gain/1
  sweep/1 -> Memory6/1
  Sum/1 -> Relational Operator/1
  Compare To Constant/1 -> Logical Operator/1
  Relational Operator/1 -> Logical Operator/2
  Constant/1 -> Sum/2
  Memory6/1 -> Sum/1

== system hapsrav_library/Cmd - Parametric/Chi Cmd/Subsystem/Azimuth angle not bounded by 0, 2pi/Counter ==
  i : Inport
  Trigger : TriggerPort  VariantControl=Variant  PortDimensions=1
  Constant : Constant
  Sum2 : Sum  Inputs=|++
  i+1 : Outport
  wires:
  i/1 -> Sum2/1
  Constant/1 -> Sum2/2
  Sum2/1 -> i+1/1

== system hapsrav_library/Cmd - Parametric/Chi Cmd/Subsystem/Azimuth angle not bounded by 0, 2pi/Counter1 ==
  i : Inport
  Trigger : TriggerPort  VariantControl=Variant  PortDimensions=1
  Constant : Constant
  Sum2 : Sum  Inputs=|+-
  i-1 : Outport
  wires:
  i/1 -> Sum2/1
  Constant/1 -> Sum2/2
  Sum2/1 -> i-1/1

== system hapsrav_library/Cmd - Parametric/Chi Cmd/Subsystem/Circular Orbit/ICs for turn ==
  t : Inport
  chi_cmd : Inport  Port=2
  Trigger : TriggerPort  VariantControl=Variant  InitialTriggerSignalState=zero
  t0 : Outport
  chi0 : Outport  Port=2
  wires:
  chi_cmd/1 -> chi0/1
  t/1 -> t0/1

== system hapsrav_library/Cmd - Parametric/Chi Cmd/Subsystem/Figure Eight Orbit/ICs for turn ==
  t : Inport
  chi : Inport  Port=2
  Trigger : TriggerPort  VariantControl=Variant  InitialTriggerSignalState=zero
  t0 : Outport
  chi0 : Outport  Port=2
  wires:
  chi/1 -> chi0/1
  t/1 -> t0/1

== system hapsrav_library/Cmd - Parametric/Chi Cmd/Subsystem/Figure Eight Orbit/Logic for figure eight following (ready==1) or initialization (ready==0) ==
  chi_cmd : Inport
  target : Inport  Port=2
  ref_axis : Inport  Port=3
  t : Inport  Port=4
  Chi Offset (when entering figure eight mode) : Subsystem
  Compare To Constant1 : simulink/Logic and Bit Operations/Compare To Constant  relop=<=  const=1*pi/180  OutDataTypeStr=boolean
  Constant : Constant  Value=2*pi
  Constant2 : Constant
  Delay1 : Delay  DelayLength=1  InitialCondition=0
  Math Function : Math  Operator=mod  SaturateOnIntegerOverflow=on
  "Start in initialization mode every time \"Figure Eight Orbit\" block is enabled. Switch to figure eight execution when angle is right." : Switch  Criteria=u2 ~= 0
  Subtract : Sum  Inputs=+-
  ready : Outport
  chi0_f8 : Outport  Port=2
  t0_f8 : Outport  Port=3
  ref0_f8 : Outport  Port=4
  wires:
  Chi Offset (when entering figure eight mode)/3(ref0_f8) -> ref0_f8/1
  Chi Offset (when entering figure eight mode)/2(t0_f8) -> t0_f8/1
  Chi Offset (when entering figure eight mode)/1(chi0_f8) -> chi0_f8/1
  t/1 -> Chi Offset (when entering figure eight mode)/3(t)
  ref_axis/1 -> Chi Offset (when entering figure eight mode)/2(ref_axis)
  target/1 -> Subtract/2
  Constant/1 -> Math Function/2
  Subtract/1 -> Math Function/1
  chi_cmd/1 -> Subtract/1, Chi Offset (when entering figure eight mode)/1(chi_cmd)
  Compare To Constant1/1 -> "Start in initialization mode every time \"Figure Eight Orbit\" block is enabled. Switch to figure eight execution when angle is right."/2
  Delay1/1 -> "Start in initialization mode every time \"Figure Eight Orbit\" block is enabled. Switch to figure eight execution when angle is right."/3
  Constant2/1 -> "Start in initialization mode every time \"Figure Eight Orbit\" block is enabled. Switch to figure eight execution when angle is right."/1
  Math Function/1 -> Compare To Constant1/1  "angle between (rad)"
  "Start in initialization mode every time \"Figure Eight Orbit\" block is enabled. Switch to figure eight execution when angle is right."/1 -> ready/1, Chi Offset (when entering figure eight mode)/Trigger, Delay1/1

== system hapsrav_library/Cmd - Parametric/Chi Cmd/Subsystem/Figure Eight Orbit/Turn at constant rate until aligned with figure eight start ==
  t : Inport
  t0 : Inport  Port=2
  chi0 : Inport  Port=3
  Gain : Gain  Gain=pi/turn_time_circle
  Subtract2 : Sum  Inputs=+-
  Sum1 : Sum  Inputs=|++
  chi_cmd : Outport
  wires:
  Sum1/1 -> chi_cmd/1
  Gain/1 -> Sum1/1
  Subtract2/1 -> Gain/1
  t0/1 -> Subtract2/2
  chi0/1 -> Sum1/2
  t/1 -> Subtract2/1

== system hapsrav_library/Cmd - Parametric/Chi Cmd/Subsystem/Racetrack Orbit/ICs for turn ==
  t : Inport
  chi : Inport  Port=2
  Trigger : TriggerPort  TriggerType=falling  VariantControl=Variant  InitialTriggerSignalState=positive
  t0 : Outport
  chi0 : Outport  Port=2
  wires:
  chi/1 -> chi0/1
  t/1 -> t0/1

== system hapsrav_library/Cmd - Parametric/Chi Cmd/Subsystem/Racetrack Orbit/Periodic Climb//Glide ==
  chi_cmd_in : Inport
  sun_az_rad : Inport  Port=2
  hold : Inport  Port=3
  0 for major-axis tracking pi/2 for minor-axis tracking : Constant  Value=rt_azimuth_offset
  Compare To Constant1 : simulink/Logic and Bit Operations/Compare To Constant  relop=<=  const=pi/4  OutDataTypeStr=boolean
  Compare To Constant2 : simulink/Logic and Bit Operations/Compare To Constant  relop=<=  const=pi/4  OutDataTypeStr=boolean
  Compare To Constant3 : simulink/Logic and Bit Operations/Compare To Constant  relop=>=  const=7*pi/4  OutDataTypeStr=boolean
  Compare To Constant4 : simulink/Logic and Bit Operations/Compare To Constant  relop=>=  const=7*pi/4  OutDataTypeStr=boolean
  Constant : Constant  Value=2*pi
  Constant1 : Constant  Value=2*pi
  Constant2 : Constant  Value=pi
  Constant3 : Constant
  Constant4 : Constant  Value=-1
  Constant5 : Constant  Value=0
  Logical Operator : Logic  AllPortsSameDT=off  OutDataTypeStr=boolean
  Logical Operator1 : Logic  AllPortsSameDT=off  OutDataTypeStr=boolean
  Logical Operator2 : Logic  Operator=OR  AllPortsSameDT=off  OutDataTypeStr=boolean
  Logical Operator3 : Logic  Operator=OR  AllPortsSameDT=off  OutDataTypeStr=boolean
  Math Function : Math  Operator=mod  SaturateOnIntegerOverflow=on
  Math Function1 : Math  Operator=mod  SaturateOnIntegerOverflow=on
  Subtract : Sum  Inputs=+--
  Subtract1 : Sum  Inputs=++--
  Switch : Switch  Criteria=u2 ~= 0
  Switch1 : Switch  Criteria=u2 ~= 0
  up_or_down : Outport
  wires:
  0 for major-axis tracking pi/2 for minor-axis tracking/1 -> Subtract/3, Subtract1/4
  Switch1/1 -> Switch/3
  Constant1/1 -> Math Function1/2
  Constant4/1 -> Switch1/1
  Constant3/1 -> Switch/1
  Constant2/1 -> Subtract1/2
  Compare To Constant3/1 -> Logical Operator2/1
  Constant5/1 -> Switch1/3
  Compare To Constant4/1 -> Logical Operator3/2
  Compare To Constant2/1 -> Logical Operator2/2
  Logical Operator1/1 -> Switch/2
  chi_cmd_in/1 -> Subtract1/1, Subtract/1
  Logical Operator/1 -> Switch1/2
  Compare To Constant1/1 -> Logical Operator3/1
  Math Function1/1 -> Compare To Constant2/1, Compare To Constant3/1
  Logical Operator2/1 -> Logical Operator1/1
  Logical Operator3/1 -> Logical Operator/2
  Subtract/1 -> Math Function/1
  Constant/1 -> Math Function/2
  sun_az_rad/1 -> Subtract1/3, Subtract/2
  Math Function/1 -> Compare To Constant1/1, Compare To Constant4/1
  Subtract1/1 -> Math Function1/1
  Switch/1 -> up_or_down/1
  hold/1 -> Logical Operator1/2, Logical Operator/1

== system hapsrav_library/Cmd - Parametric/Chi Cmd/Subsystem/Racetrack Orbit/Pulsing Logic: 1 for hold course 0 for turn ==
  t : Inport
  chi : Inport  Port=2
  sun_az_rad : Inport  Port=3
  last_chi : Inport  Port=4
  0 for major-axis tracking pi/2 for minor-axis tracking : Constant  Value=rt_azimuth_offset
  Compare To Constant : simulink/Logic and Bit Operations/Compare To Constant  relop=<=  const=hold_time  OutDataTypeStr=boolean
  Compare To Constant1 : simulink/Logic and Bit Operations/Compare To Constant  relop=<=  const=1*pi/180  OutDataTypeStr=boolean
  Compare To Constant2 : simulink/Logic and Bit Operations/Compare To Constant  relop=>=  const=10*pi/180  OutDataTypeStr=boolean
  Compare To Constant3 : simulink/Logic and Bit Operations/Compare To Constant  relop=>  const=1  OutDataTypeStr=boolean
  Compare To Constant4 : simulink/Logic and Bit Operations/Compare To Constant  relop=<=  const=350*pi/180  OutDataTypeStr=boolean
  Constant : Constant  Value=pi
  Constant1 : Constant  Value=2*pi
  Constant2 : Constant  Value=0
  "Initial condition: Start by turning, if required" : Switch  Criteria=u2 ~= 0
  Logical Operator : Logic  AllPortsSameDT=off  OutDataTypeStr=boolean
  Logical Operator1 : Logic  AllPortsSameDT=off  OutDataTypeStr=boolean
  Math Function : Math  Operator=mod  SaturateOnIntegerOverflow=on
  Math Function1 : Math  Operator=mod  SaturateOnIntegerOverflow=on
  Scope : Scope  NumInputPorts=3
  Subtract : Sum  Inputs=+-
  Subtract1 : Sum  Inputs=+-
  Subtract2 : Sum  Inputs=+-
  Sum1 : Sum  Inputs=|++
  timer : Subsystem  TreatAsAtomicUnit=on
  hold (bool) : Outport
  wires:
  Compare To Constant2/1 -> Logical Operator1/1
  Compare To Constant4/1 -> Logical Operator1/2
  Compare To Constant3/1 -> "Initial condition: Start by turning, if required"/2
  Constant2/1 -> "Initial condition: Start by turning, if required"/3
  Compare To Constant/1 -> "Initial condition: Start by turning, if required"/1
  0 for major-axis tracking pi/2 for minor-axis tracking/1 -> Sum1/2
  sun_az_rad/1 -> Sum1/1
  Compare To Constant1/1 -> Logical Operator/1, Scope/2
  Logical Operator1/1 -> Scope/3, Logical Operator/2
  last_chi/1 -> Subtract2/2
  chi/1 -> Subtract2/1, Subtract/1
  Constant1/1 -> Math Function1/2
  Math Function1/1 -> Compare To Constant2/1, Compare To Constant4/1  "angle between current and last hold (make sure turn isn't just a couple degrees)"
  Subtract2/1 -> Math Function1/1
  Sum1/1 -> Subtract/2
  t/1 -> timer/1(t), Subtract1/1
  Constant/1 -> Math Function/2
  Subtract1/1 -> Compare To Constant/1, Scope/1
  Logical Operator/1 -> timer/Trigger  "trigger right direction"
  Subtract/1 -> Math Function/1
  "Initial condition: Start by turning, if required"/1 -> hold (bool)/1
  Math Function/1 -> Compare To Constant1/1  "angle between (rad)"
  timer/1(t0) -> Subtract1/2, Compare To Constant3/1

== system hapsrav_library/Cmd - Parametric/Chi Cmd/Subsystem/Racetrack Orbit/Turn at constant rate ==
  t : Inport
  t0 : Inport  Port=2
  chi0 : Inport  Port=3
  Gain : Gain  Gain=pi/turn_time_rt
  Subtract2 : Sum  Inputs=+-
  Sum1 : Sum  Inputs=|++
  chi_cmd : Outport
  wires:
  Sum1/1 -> chi_cmd/1
  Gain/1 -> Sum1/1
  Subtract2/1 -> Gain/1
  t0/1 -> Subtract2/2
  chi0/1 -> Sum1/2
  t/1 -> Subtract2/1

== system hapsrav_library/hapsrav_main/Kinematic 6DOF/Aero/CL vs AoA/CD LUT ==
  alpha : Inport
  alt : Inport  Port=2
  0 <= Alt <= 24575 : Saturate  UpperLimit=max_alt_bp  LowerLimit=min_alt_bp
  CD LUT : Lookup_n-D  BreakpointsForDimension1=alpha_bp  BreakpointsForDimension2=alt_bp  BeginIndexSearchUsingPreviousIndexResult=on  Table=cd_data  ExtrapMethod=Clip  RemoveProtectionInput=on  UseLastTableValue=on  InternalRulePriority=Speed  RndMeth=Simplest  InputSameDT=on
  aoa_min <= alpha <= aoa_max : Saturate  UpperLimit=max_alpha_bp  LowerLimit=min_alpha_bp
  CD : Outport
  wires:
  CD LUT/1 -> CD/1
  alt/1 -> 0 <= Alt <= 24575/1
  0 <= Alt <= 24575/1 -> CD LUT/2
  alpha/1 -> aoa_min <= alpha <= aoa_max/1
  aoa_min <= alpha <= aoa_max/1 -> CD LUT/1
